simulink model "Zadanie_2"  (Simulink 7.1)
settings: Solver=ode45  StartTime=0.0  StopTime=1  RelTol=1e-3
settings Model: Creator=Michal  LastModifiedBy=Michal

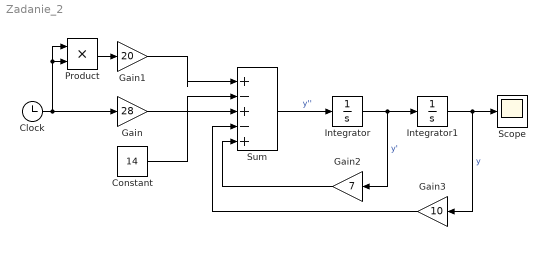
== system Zadanie_2 ==
  Clock : Clock
      settings: Decimation=10
  Constant : Constant  Value=14  OutDataType=sfix(16)  OutScaling=2^0
  Gain : Gain  Gain=28  ParameterDataType=sfix(16)  ParameterScaling=2^0  OutDataType=sfix(16)  OutScaling=2^0
  Gain1 : Gain  Gain=20  ParameterDataType=sfix(16)  ParameterScaling=2^0  OutDataType=sfix(16)  OutScaling=2^0
  Gain2 : Gain  Orientation=left  Gain=7  ParameterDataType=sfix(16)  ParameterScaling=2^0  OutDataType=sfix(16)  OutScaling=2^0
  Gain3 : Gain  Orientation=left  Gain=10  ParameterDataType=sfix(16)  ParameterScaling=2^0  OutDataType=sfix(16)  OutScaling=2^0
  Integrator : Integrator
  Integrator1 : Integrator
  Product : Product  OutDataType=sfix(16)  OutScaling=2^0  RndMeth=Zero
  Scope : Scope
  Sum : Sum  Inputs=|+-+-+  OutDataType=sfix(16)  OutScaling=2^0
  wires:
  Clock/1 -> Gain/1, Product/2, Product/1
  Product/1 -> Gain1/1
  Gain1/1 -> Sum/1
  Gain/1 -> Sum/2
  Constant/1 -> Sum/3
  Sum/1 -> Integrator/1  "y''"
  Integrator/1 -> Integrator1/1, Gain2/1  "y'"
  Integrator1/1 -> Scope/1, Gain3/1  "y"
  Gain3/1 -> Sum/4
  Gain2/1 -> Sum/5
